simulink model "ex9"  (R2018a)
settings: Solver=VariableStepAuto  StartTime=0.0  StopTime=0.033  RelTol=1e-3
libraries: powerlib x9, powerlib_meascontrol x1
settings Model: Creator=Asus  LastModifiedBy=Asus

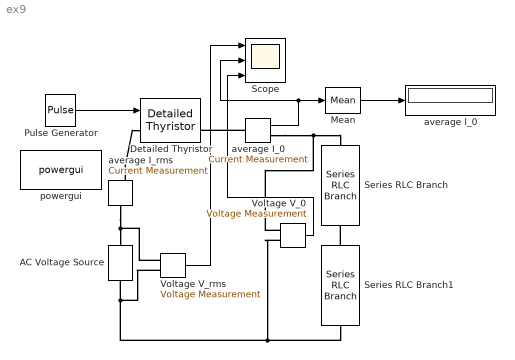
== system ex9 ==
  AC Voltage Source : powerlib/Electrical Sources/AC Voltage Source  Amplitude=120*sqrt(2)  Phase=0  Frequency=60  SampleTime=0  Measurements=None  BusType=swing  Pref=10e3  Qref=0  Qmin=-inf  Qmax=+inf
  Detailed Thyristor : powerlib/Power Electronics/Detailed Thyristor  Ron=0.001  Lon=1e-3  Vf=0.8  IL=0.1  Tq=100e-6  IC=0  Rs=500  Cs=250e-9  Measurements=on
      settings: SourceProductName=Simscape Power Systems  SourceProductBaseCode=PS
  Mean : powerlib_meascontrol/Measurements/Mean  Freq=60  Vinit=0  Ts=0
  Pulse Generator : DiscretePulseGenerator  PulseType=Time based  Period=0.0166  PulseWidth=10  PhaseDelay=35/(120*180)
  Scope : Scope  NumInputPorts=3
  Series RLC Branch : powerlib/Elements/Series RLC Branch  LConnTagsString=__new0  RConnTagsString=__new0  BranchType=R  Resistance=20  Inductance=1e-3  SetiL0=off  InitialCurrent=0  Capacitance=1e-6  Setx0=off  InitialVoltage=0  Measurements=None
  Series RLC Branch1 : powerlib/Elements/Series RLC Branch  LConnTagsString=__new0  RConnTagsString=__new0  BranchType=L  Resistance=30  Inductance=0.04  SetiL0=off  InitialCurrent=0  Capacitance=1e-6  Setx0=off  InitialVoltage=0  Measurements=None
  Voltage V_0 : powerlib/Measurements/Voltage Measurement  PhasorSimulation=off  OutputType=Complex  PSBequivalent=0
  Voltage V_rms : powerlib/Measurements/Voltage Measurement  PhasorSimulation=off  OutputType=Complex  PSBequivalent=0
  average I_0 : Display
  "average I_0 " : powerlib/Measurements/Current Measurement  PhasorSimulation=off  OutputType=Complex  PSBequivalent=0
  "average I_rms " : powerlib/Measurements/Current Measurement  PhasorSimulation=off  OutputType=Complex  PSBequivalent=0
  powergui : powerlib/powergui  Priority=1  SimulationMode=Continuous  SampleTime=50e-6  frequency=60  Iterations=50  frequencyindice=0  Pbase=100e6  ErrMax=1e-4  UnitsV=kV  UnitsW=MW  buscounter=0  FunctionMessages=off  echomessages=off  EnableUseOfTLC=off  CurrentSourceSwitches=off  DisableSnubberDevices=off  DisableRonSwitches=off  DisableVfSwitches=off  DisplayEquations=off  SolverType=Tustin/Backward Euler (TBE)  Interpol=off  ExternalGateDelay=off  methode=off  Ts=100  x0status=blocks  SPID=on  SwTol=0  HookPort=off  RestoreLinks=warning  ResistiveCurrentMeasurement=off  Frange=[0:2:500]  Ylog=off  Xlog=on  ShowGrid=off  save=off  variable=ZData  structure=0  ZoomFFT=off  StartTime=0.0  cycles=1  DisplayStyle=1  fundamental=60  FreqAxis=off  MaxFrequency=1000  frequencyindicesteady=1  RmsSteady=1  display=off
  wires:
  Pulse Generator/1 -> Detailed Thyristor/1
  Voltage V_rms/1 -> Scope/1
  Mean/1 -> average I_0/1
  Voltage V_0/1 -> Scope/3
  "average I_0 "/1 -> Scope/2, Mean/1
  connections:
  Voltage V_rms/LConn2 -- Voltage V_0/LConn2 -- Series RLC Branch1/RConn1 -- AC Voltage Source/LConn1
  "average I_0 "/RConn1 -- Series RLC Branch/LConn1 -- Voltage V_0/LConn1
  AC Voltage Source/RConn1 -- "average I_rms "/LConn1 -- Voltage V_rms/LConn1
  "average I_rms "/RConn1 -- Detailed Thyristor/LConn1
  "average I_0 "/LConn1 -- Detailed Thyristor/RConn1
  Series RLC Branch1/LConn1 -- Series RLC Branch/RConn1
